simulink model "PID_controller"  (R2020b)
settings: Solver=VariableStepAuto  StartTime=0.0  StopTime=10  RelTol=1e-3
values from neighbouring files (symbols this model uses):
  kd = 6.98    [position_data.sldd]
  ki = 12396450.7067    [position_data.sldd]
  kp = 18842.98    [position_data.sldd]
settings Model: DataDictionary=position_data.sldd  Creator=Ravi  LastModifiedBy=Ravi
settings DataIOCC: SaveOutput=off  SaveTime=off

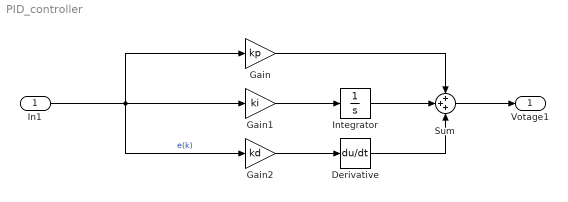
== system PID_controller ==
  In1 : Inport  OutDataTypeStr=double  PortDimensions=1  SampleTime=0
  Derivative : Derivative
  Gain : Gain  Gain=kp
  Gain1 : Gain  Gain=ki
  Gain2 : Gain  Gain=kd
  Integrator : Integrator
  Sum : Sum  Inputs=+++
  Votage1 : Outport  OutDataTypeStr=double  PortDimensions=1  SampleTime=0
  wires:
  In1/1 -> Gain1/1, Gain2/1, Gain/1  "e(k)"
  Derivative/1 -> Sum/3
  Gain2/1 -> Derivative/1
  Gain/1 -> Sum/1
  Gain1/1 -> Integrator/1
  Integrator/1 -> Sum/2
  Sum/1 -> Votage1/1
